simulink model "MF_artigo_Roberta"  (R2013b)
settings: Solver=ode45  StartTime=0.0  StopTime=.15  RelTol=1e-3
libraries: dsparch4 x1
settings Model: Creator=Roberta Martin  LastModifiedBy=Roberta
settings ConfigurationSet: Description=SimMechanics 2G

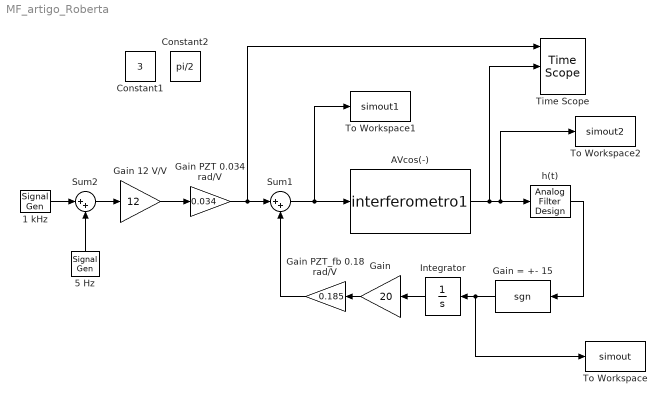
== system MF_artigo_Roberta ==
  " 5 Hz" : SignalGenerator  Amplitude=3  Frequency=5
  "1 kHz " : SignalGenerator  Amplitude=1.5  Frequency=1000
  AVcos(-) : M-S-Function  FunctionName=interferometro1
  Constant1 : Constant  Value=3
  Constant2 : Constant  Value=pi/2
  Gain : Gain  Gain=20
  Gain 12 V/V : Gain  Gain=12
  Gain = +- 15 : M-S-Function  FunctionName=sgn
  Gain PZT 0.034 rad/V : Gain  Gain=0.034
  Gain PZT_fb 0.18 rad/V : Gain  Gain=0.185
  Integrator : Integrator  LimitOutput=on  UpperSaturationLimit=15  LowerSaturationLimit=-15
  Sum1 : Sum  Inputs=|++
  Sum2 : Sum  Inputs=|++
  Time Scope : TimeScope  NumInputPorts=3  DefaultConfigurationName=spbscopes.TimeScopeBlockCfg
      settings: CopyFcn=scopeextensions.ScopeBlock.onCoreBlockCopy(gcbh);  DeleteFcn=scopeextensions.ScopeBlock.callback(gcbh, 'onBlockDelete');  PreSaveFcn=scopeextensions.ScopeBlock.callback(gcbh, 'onModelSave');  NameChangeFcn=scopeextensions.ScopeBlock.callback(gcbh, 'onBlockRename');  DestroyFcn=scopeextensions.ScopeBlock.onBlockDestroy(gcbh)  OpenFcn=scopeextensions.SrcWiredSL.coreBlockCommand('Open',gcbh)  CloseFcn=scopeextensions.ScopeBlock.callback(gcbh, 'onBlockClose');  PreDeleteFcn=scopeextensions.ScopeBlock.callback(gcbh, 'onBlockPreDelete');
  To Workspace : ToWorkspace  VariableName=simout  SampleTime=-1  SaveFormat=Structure With Time
  To Workspace1 : ToWorkspace  VariableName=simout1  SampleTime=-1  SaveFormat=Structure With Time
  To Workspace2 : ToWorkspace  VariableName=simout2  SampleTime=-1  SaveFormat=Structure With Time
  h(t) : dsparch4/Analog Filter Design  method=Butterworth  filttype=Lowpass  N=1  Wlo=20*2*pi()  Whi=80  Rp=2  Rs=40
  wires:
  AVcos(-)/1 -> Time Scope/2, To Workspace2/1, h(t)/1
  Sum1/1 -> To Workspace1/1, AVcos(-)/1
  Gain/1 -> Gain PZT_fb 0.18 rad/V/1
  Gain PZT 0.034 rad/V/1 -> Time Scope/1, Sum1/1
  Gain 12 V/V/1 -> Gain PZT 0.034 rad/V/1
  Sum2/1 -> Gain 12 V/V/1
  Gain PZT_fb 0.18 rad/V/1 -> Sum1/2
  "1 kHz "/1 -> Sum2/1
  h(t)/1 -> Gain = +- 15/1
  Gain = +- 15/1 -> To Workspace/1, Integrator/1
  Integrator/1 -> Gain/1
  " 5 Hz"/1 -> Sum2/2
